simulink model "RobotX_FullSystemSep20"  (R2014a)
settings: Solver=FixedStepDiscrete  StartTime=0.0  StopTime=inf  FixedStep=.25  RelTol=1e-3
undefined symbols (not defined in the file): Com1, Com2, Com3, Com4, DiscIntNeverNeededParam, standard
libraries: simulink x11, xpcseriallib x11, slrtlib x3, speedgoatlib x1, speedgoatlib_IO102 x1
(part 2 of 4)

== matlab function RobotX_FullSystemSep20/Main FSM/Start//Speedgate/Start Gate/Calculate Times ==
  data: pts input; u input; Data output
function Data = calcTimes(pts, u)
%Written by Anderson Lebbad on August 9, 2014
%Last Edited:

%Calculates times for the boat to get to points for a trajectory, and
%formats Data for communication

%Initialize
Data = zeros(24,1);
traj = zeros(8,3);

pts8 = [pts(1,:); (pts(2,:)-pts(1,:))/3; 2*(pts(2,:)-pts(1,:))/3; pts(2,:);...
    (pts(3,:)-pts(2,:))/2; pts(3,:); (pts(4,:)-pts(3,:))/2; pts(4,:)];

traj(:,1:2) = pts8;

for k = 2:8
    %Calculate distance to travel from last point
    distTravel = sqrt(sum((pts8(k-1,:)-pts8(k,:)).^2));
    %Assume 1m per second speed
    traj(k,3) = traj(k-1,3) + distTravel;
    %Add time based off initial velocity to get to first point past initial
    if k == 2
        traj(k,3) = traj(k,3) + 2.5*abs(2-u);
    end
end


%Output Data
for i=1:8
    for j = 1:3
        Data(3*(i-1)+j) = traj(i,j);
    end
end

== matlab function RobotX_FullSystemSep20/Main FSM/Start//Speedgate/Start Gate/Gate ==
  data: HeldHeading input; Finished output; Valid output; X input; Y input; Psi input; Dist input; Angles input; pts output; idx input
function [Finished, Valid, pts] = Gate(HeldHeading,X,Y,Psi,Dist,Angles,idx)
%Written by Anderson Lebbad on August 9, 2014
%Last Edited by:

%This function sends a forward trajectory (from the initial heading read
%into it) until a landmark is found. Once the landmark is found, a
%trajectory is written to dodge around it.

persistent Found finPt sample
if isempty(Found)
    Found = 0;
    finPt = [0 0];
    sample = 50;
end

dodgeLength = 15;
dodgeWidth = 5;
Finished = 0;
Valid = 0;
pts = zeros(4,2);
%Distance to object in meters
DistM = Dist/100;

%Set Valid bit. If it has been found in a previous timestep, the point is
%invalid, otherwise it is valid every increment of ts or if an object is
%found

%If no Landmark is found, navigate forward
if Found == 0
    %Initial pt
    pts(1,1) = X + 5*cos(HeldHeading*pi/180);
    pts(1,2) = Y + 5*sin(HeldHeading*pi/180);
    %Nothing found
    if idx(1) == 0
        pts(2,1) = X + 10*cos(HeldHeading*pi/180);
        pts(2,2) = Y + 10*sin(HeldHeading*pi/180);
        pts(3,1) = X + 15*cos(HeldHeading*pi/180);
        pts(3,2) = Y + 15*sin(HeldHeading*pi/180);
        pts(4,1) = X + 20*cos(HeldHeading*pi/180);
        pts(4,2) = Y + 20*sin(HeldHeading*pi/180);
        %Only flip valid bit every ts (seconds)
        sample = sample + 1;
        if sample >= 50
            Valid = 1;
            sample = 0;
        end
        %Something found
    elseif idx(2) == 0
        %Absolute Heading of object relative to boat's position
        landmarkHeading = mod((Psi + Angles(idx(1))),360);
        lmHeadingRad = landmarkHeading*pi/180;
        %Navigate to it
        pts(2,1) = X + DistM(idx(1))*cos(lmHeadingRad) - dodgeWidth*sin(lmHeadingRad);
        pts(2,2) = Y + DistM(idx(1))*sin(lmHeadingRad) + dodgeWidth*cos(lmHeadingRad);
        pts(3,1) = X + (DistM(idx(1)) + dodgeLength)*cos(lmHeadingRad);
        pts(3,2) = Y + (DistM(idx(1)) + dodgeLength)*sin(lmHeadingRad);
        pts(4,1) = X + (DistM(idx(1)) + 2*dodgeLength)*cos(lmHeadingRad);
        pts(4,2) = Y + (DistM(idx(1)) + 2*dodgeLength)*sin(lmHeadingRad);
        finPt = pts(4,:);
        %Flip valid if found
        Valid = 1;
        %Tag object as having been found
        Found = 1;
    else
        %Absolute Heading of object relative to boat's position
        landmarkHeading1 = mod((Psi + Angles(idx(1))),360);
        lmHeadingRad1 = landmarkHeading1*pi/180;
        landmarkHeading2 = mod((Psi + Angles(idx(2))),360);
        lmHeadingRad2 = landmarkHeading2*pi/180;
        %Landmark locations in NED
        lmX1 = X + DistM(idx(1))*cos(lmHeadingRad1);
        lmY1 = Y + DistM(idx(1))*sin(lmHeadingRad1);
        lmX2 = X + DistM(idx(2))*cos(lmHeadingRad2);
        lmY2 = Y + DistM(idx(2))*sin(lmHeadingRad2);
        %Middle point
        midX = (lmX1 + lmX2) / 2;
        midY = (lmY1 + lmY2) / 2;
        %Navigate to it
        pts(2,1) = midX;
        pts(2,2) = midY;
        %Hold heading and continue from midpoint
        pts(3,1) = midX + 5*cos(HeldHeading*pi/180);
        pts(3,2) = midY + 5*sin(HeldHeading*pi/180);
        pts(4,1) = midX + 10*cos(HeldHeading*pi/180);
        pts(4,2) = midY + 10*sin(HeldHeading*pi/180);
        finPt = pts(4,:);
        %Flip valid if found
        Valid = 1;
        %Tag object as having been found
        Found = 2;
    end
end

if Found == 1
    if idx(2) ~= 0
        %Absolute Heading of object relative to boat's position
        landmarkHeading1 = mod((Psi + Angles(idx(1))),360);
        lmHeadingRad1 = landmarkHeading1*pi/180;
        landmarkHeading2 = mod((Psi + Angles(idx(2))),360);
        lmHeadingRad2 = landmarkHeading2*pi/180;
        %Landmark locations in NED
        lmX1 = X + DistM(idx(1))*cos(lmHeadingRad1);
        lmY1 = Y + DistM(idx(1))*sin(lmHeadingRad1);
        lmX2 = X + DistM(idx(2))*cos(lmHeadingRad2);
        lmY2 = Y + DistM(idx(2))*sin(lmHeadingRad2);
        %Middle point
        midX = (lmX1 + lmX2) / 2;
        midY = (lmY1 + lmY2) / 2;
        %Navigate to it
        pts(2,1) = midX;
        pts(2,2) = midY;
        %Hold heading and continue from midpoint
        pts(3,1) = midX + 5*cos(HeldHeading*pi/180);
        pts(3,2) = midY + 5*sin(HeldHeading*pi/180);
        pts(4,1) = midX + 10*cos(HeldHeading*pi/180);
        pts(4,2) = midY + 10*sin(HeldHeading*pi/180);
        finPt = pts(4,:);
        %Flip valid if found
        Valid = 1;
        %Tag object as having been found
        Found = 2;
    end
end

%Check to see how far the current pose is from the final point in the
%trajectory
if Found >= 1
range = abs(finPt(1)-X)+abs(finPt(2)-Y);
else
    range = 1000;
end
if range <= 5
    Finished = 1;
end

end

== matlab function RobotX_FullSystemSep20/Main FSM/Acoustic FSM/Drive Pt1/CalcTimes ==
  data: pts input; u input; Data output
function Data = calcTimes(pts, u)
%Written by Anderson Lebbad on August 9, 2014
%Last Edited: Dylan DeGaetano September 1, 2014

%Calculates times for the boat to get to points for a trajectory, and
%formats Data for communication

%Initialize
Data = zeros(24,1);
traj = zeros(8,3);
traj(:,1:2) = pts;



for k = 2:8
    %Calculate distance to travel from last point
    distTravel = sqrt(sum((pts(k-1,:)-pts(k,:)).^2));
    %Assume 1m per second speed
    traj(k,3) = traj(k-1,3) + distTravel;
    %Add time based off initial velocity to get to first point past initial
    if k == 2
        traj(k,3) = traj(k,3) + 2.5*abs(2-u);
    end
end


%Output Data
for i=1:8
    for j = 1:3
        Data(3*(i-1)+j) = traj(i,j);
    end
end

== matlab function RobotX_FullSystemSep20/Main FSM/Light Beacon/Approach/CalcTimes ==
  data: pts input; u input; Data output
function Data = calcTimes(pts, u)
%Written by Anderson Lebbad on August 9, 2014
%Last Edited: Dylan DeGaetano September 1, 2014

%Calculates times for the boat to get to points for a trajectory, and
%formats Data for communication

%Initialize
Data = zeros(24,1);
traj = zeros(8,3);
traj(:,1:2) = pts;



for k = 2:8
    %Calculate distance to travel from last point
    distTravel = sqrt(sum((pts(k-1,:)-pts(k,:)).^2));
    %Assume 1m per second speed
    traj(k,3) = traj(k-1,3) + distTravel;
    %Add time based off initial velocity to get to first point past initial
    if k == 2
        traj(k,3) = traj(k,3) + 2.5*abs(2-u);
    end
end


%Output Data
for i=1:8
    for j = 1:3
        Data(3*(i-1)+j) = traj(i,j);
    end
end

== matlab function RobotX_FullSystemSep20/Main FSM/Acoustic FSM/Drive Pt1/GPSMove ==
  data: X input; Finished output; valid output; Y input; Psi input; GoalPt input; pts output
function [Finished, valid, pts] = GPSmove(X,Y,Psi,GoalPt)
%Written by Dylan DeGaetano on September 1, 2014
%Last edited by: Michael Benson on September 4, 2014
%   Changed Sample to be a persistent variable so that pts will not be
%   recalculated every iteration.
%
%This function will go to a given NED cooridnate 



persistent Sample

if isempty(Sample)
    Sample = 0;
end

valid = 0;
Finished = 0;
pts = zeros(8,2);
%$Distance to object in meters

if Sample == 0
    valid = 1;
    pts(1,1) = X+5*cos(Psi*pi/180);
    pts(1,2) = Y+5*cos(Psi*pi/180);
    pts(8,1) = GoalPt(1,1);
    pts(8,2) = GoalPt(1,2);
    pts(2,:) = pts(1,:) +(1*(GoalPt-pts(1,:))/7);
    pts(3,:) = pts(1,:) +(2*(GoalPt-pts(1,:))/7);
    pts(4,:) = pts(1,:) +(3*(GoalPt-pts(1,:))/7);
    pts(5,:) = pts(1,:) +(4*(GoalPt-pts(1,:))/7);
    pts(6,:) = pts(1,:) +(5*(GoalPt-pts(1,:))/7);
    pts(7,:) = pts(1,:) +(6*(GoalPt-pts(1,:))/7);
    Sample = 1; 
else 
    range = sqrt(sum((GoalPt - [X Y]).^2));
    if range <= 3
        Finished = 1;
    end
end

== matlab function RobotX_FullSystemSep20/Main FSM/Light Beacon/Light Enabler ==
  data: taskSelector output; quadOut output; GPSEn output; SpinEn output; ApprchEn output; StareEn output; mainTask input; GPSFin input; SpinFin input; ApprchFin input; Found input
function [taskSelector,quadOut,GPSEn,SpinEn,ApprchEn,StareEn]=...
    Light_Enabler(mainTask,GPSFin,SpinFin,ApprchFin,Found)
%Written by Anderson Lebbad on July 19, 2013
%Last Edited: Dylan DeGaetano on September ,8 2014
%   Substring search for task was written in
%   Case switches were redundant, combined with first set of if statements
%
%Changes the value of MainMode and the enablers for the tasks within the
%Light Beacon FSM.
%Will loop through move and spin commands 5 times before terminating if
%nothing is found
persistent quad

if isempty (quad)
    quad = 0;
end


% Initialize enable signals
GPSEn = 0;
SpinEn = 0;
StareEn = 0;
ApprchEn = 0;

% Convert main task indicator to a string
mainTaskStr = char(mainTask);

% Adjust finished states based on user task selection (never skips
% initialization)
if ~isempty(strfind(mainTaskStr,'spin'))
    GPSFin = 1;
elseif ~isempty(strfind(mainTaskStr,'stare'))
    Found = 1;
end

%adjust finish states based on interation through loop
if (GPSFin == 1)&&(SpinFin == 1)&&(quad <=4)
    GPSFin = 0;
    quad = quad +1;
end

% Set enable signals based on state completion
if ApprchFin == 1;
    StareEn = 1;
    taskSelector = 4;
elseif Found == 1;
    ApprchEn = 1;
    taskSelector = 3;
elseif GPSFin == 0
    GPSEn = 1;
    taskSelector = 1;
else
    SpinEn = 1;
    taskSelector = 2;
end

quadOut = quad;

== matlab function RobotX_FullSystemSep20/Main FSM/Light Beacon/Stare/MATLAB Function ==
  data: X input; Data output; Y input; Psi input; Angles input; idx input; LidarMode output
function [Data,LidarMode] = Orient(X,Y,Psi,Angles,idx)
%Written by Dylan DeGaetano on September 2, 2014
%Last Edited:Dylan DeGaetano on September 10,2014

%This function passes the current pose data added to the angle of the Light 
%buoy This stare forces the Boat to stare at the bouy.This task must be in station 
%keeping mode

persistent holdPose Locked

if isempty(holdPose)
    holdPose = [X Y Psi];
    Locked = 0;
end

if Locked == 0
    if idx(1) ~= 0
        holdPose(3) = Psi + Angles(idx(1));
        Locked = 1;
    end
end

%Initialize Data variable
Data = zeros(24,1);

%Set desired pose
Data(1) = holdPose(1);
Data(2) = holdPose(2);
Data(3) = holdPose(3);

if Locked == 0
    LidarMode = 1;
else
    LidarMode = 7;
end

end

== matlab function RobotX_FullSystemSep20/Main FSM/Light Beacon/GPS Move/CalcTimes ==
  data: pts input; u input; Data output
function Data = calcTimes(pts, u)
%Written by Anderson Lebbad on August 9, 2014
%Last Edited: Dylan DeGaetano September 1, 2014

%Calculates times for the boat to get to points for a trajectory, and
%formats Data for communication

%Initialize
Data = zeros(24,1);
traj = zeros(8,3);
traj(:,1:2) = pts;



for k = 2:8
    %Calculate distance to travel from last point
    distTravel = sqrt(sum((pts(k-1,:)-pts(k,:)).^2));
    %Assume 1m per second speed
    traj(k,3) = traj(k-1,3) + distTravel;
    %Add time based off initial velocity to get to first point past initial
    if k == 2
        traj(k,3) = traj(k,3) + 2.5*abs(2-u);
    end
end


%Output Data
for i=1:8
    for j = 1:3
        Data(3*(i-1)+j) = traj(i,j);
    end
end

== matlab function RobotX_FullSystemSep20/Main FSM/Light Beacon/GPS Move/GPSMove ==
  data: GoalN input; GoalE input; X input; Finished output; valid output; Y input; Psi input; pts output
function [Finished,valid,pts] = GPSmove(GoalN,GoalE,X,Y,Psi)
%Written by Dylan DeGaetano on September 1, 2014
%Last edited by: Anderson Lebbad
%
%This function will go to a given NED cooridnate, last edit changed the
%goal pt and variable names

GoalNED = [GoalN GoalE];

persistent Sample
if isempty(Sample)
Sample = 0;
end
Finished = 0;
pts = zeros(8,2);
%$Distance to object in meters

if Sample == 0
    pts(1,1) = X+5*cos(Psi*pi/180);
    pts(1,2) = Y+5*cos(Psi*pi/180);
    pts(8,:) = GoalNED;
    pts(2,:) = pts(1,:) +(1*(GoalNED-pts(1,:))/7);
    pts(3,:) = pts(1,:) +(2*(GoalNED-pts(1,:))/7);
    pts(4,:) = pts(1,:) +(3*(GoalNED-pts(1,:))/7);
    pts(5,:) = pts(1,:) +(4*(GoalNED-pts(1,:))/7);
    pts(6,:) = pts(1,:) +(5*(GoalNED-pts(1,:))/7);
    pts(7,:) = pts(1,:) +(6*(GoalNED-pts(1,:))/7);
    Sample = 1; 
    valid = 1;
    
else 
    range = sqrt(sum((GoalNED - [X Y]).^2));
    if range <= 5
        Finished = 1;
    end
    valid = 0;
end

== matlab function RobotX_FullSystemSep20/Main FSM/Light Beacon/GPS Move/LLA to NED ==
  data: quad input; GoalLLA input; GoalN output; NED_origin input; GoalE output
function [GoalN, GoalE]  = LLA2NED(quad,GoalLLA,NED_origin)
%Written by Anderson Lebbad on September 20, 2014
%Last edited by:
%
%This function converts a target Latitude, Longitude, Altitude (LLA) point
%into North, East, Down (NED) coordinates

%First convert to earth centered, earth fixed frame
if quad == 0
    TargetLLA = sum(GoalLLA)./4;
else
    TargetLLA = GoalLLA(quad,:);
end

GoalECEF = lla2ecef([TargetLLA(1); TargetLLA(2); 0]);
%Then convert from ECEF to North East Down
GoalNEDvect = ecef2ned(NED_origin,GoalECEF);
GoalN = GoalNEDvect(1);
GoalE = GoalNEDvect(2);

end

function x_ecef = lla2ecef(x_lla)
% LLE2ECEF: Converts from geodetic latitude, longitude, and altitude to earth-centered earth-fixed Cartesian coordinates
% INPUT: latitude phi (rad), longitude lambda (rad), altitude h (m)
% OUTPUT: [x, y, z]' (m) earth-centered earth-fixed Cartesian coordinates
    a = 6378137; % equatorial radius of ellipsoid (semi-major axis) (m)
    b = 6356752; % polar axis radius of ellipsoid (semi-minor axis) (m)

    phi = x_lla(1);
    lambda = x_lla(2);
    h = x_lla(3);
    
    % auxiliar quantities f, e, and N
    f = (a-b)/a;
    e = f*(2-f);
    N = a/sqrt(1-(e*sin(phi))^2);
    x_ecef = [(N+h)*cos(phi)*cos(lambda); (N+h)*cos(phi)*sin(lambda); (N*(1-e^2)+h)*sin(phi)];
end

function [x_ned] = ecef2ned(ned_lla, x_ecef)
% ECEF2NED Converts from earth-centered, earth-fixed Cartesian coordinates to tangent plane
% INPUT:
% 1) x_ecef=[x,y,z]' (m) earth-centered, earth-fixed Cartesian coordinates
% 2) ned_lla=[phi,lambda]' consiting of latitude phi (rad), longitude lambda (rad) of NED origin
% OUTPUT:
% 1) x_ned=[x,y,z]' (m) in NED coordinate system with the origin [phi,lambda]'

    phi = ned_lla(1);
    lambda = ned_lla(2);

    % transformation  matrix
    T = [-sin(phi)*cos(lambda) -sin(phi)*sin(lambda)  cos(phi)
         -sin(lambda)           cos(lambda)           0
          cos(phi)*cos(lambda)   cos(phi)*sin(lambda)  sin(phi)];

     x_ned = T*(x_ecef-lla2ecef([phi, lambda, 0]')); % convert to NED
     x_ned(3) = -x_ned(3);
end

== matlab function RobotX_FullSystemSep20/Main FSM/Acoustic FSM/Main Enabler ==
  data: taskSelector output; Drive1En output; Acoustic1En output; Drive2En output; Drive1Fin input; Acoustic1Fin input; Drive2Fin input; Acoustic2Fin input; Drive3Fin input; Acoustic3Fin input; Acoustic2En output; Drive3En output; Acoustic3En output; PointEn output
function [taskSelector,Drive1En,Acoustic1En,Drive2En,Acoustic2En,Drive3En,...
    Acoustic3En,PointEn] = taskEnabler(Drive1Fin,Acoustic1Fin,Drive2Fin,...
    Acoustic2Fin,Drive3Fin,Acoustic3Fin)
%Written by Anderson Lebbad on July 19, 2013
%Last Edited: Edward Zhu on June 2, 2014
%   Substring search for task was written in
%   Case switches were redundant, combined with first set of if statements

%Changes the value of MainMode and the enablers for the tasks within the
%Main FSM.

% Initialize enable signals
Drive1En = 0;
Acoustic1En = 0;
Drive2En = 0;
Acoustic2En = 0;
Drive3En = 0;
Acoustic3En = 0;
PointEn = 0;

% Set enable signals based on state completion
if Drive1Fin == 0
    Drive1En = 1;
    taskSelector = 1;
elseif Acoustic1Fin == 0
    Acoustic1En = 1;
    taskSelector = 2;
elseif Drive2Fin == 0
    Drive2En = 1;
    taskSelector = 3;
elseif Acoustic2Fin == 0
    Acoustic2En = 1;
    taskSelector = 4;
elseif Drive3Fin == 0
    Drive3En = 1;
    taskSelector = 5;
elseif Acoustic3Fin == 0
    Acoustic3En = 1;
    taskSelector = 6;
else
    PointEn = 1;
    taskSelector = 7;
end

== matlab function RobotX_FullSystemSep20/Main FSM/Termination/CalcTimes ==
  data: pts input; u input; Data output
function Data = calcTimes(pts, u)
%Written by Anderson Lebbad on August 9, 2014
%Last Edited: Dylan DeGaetano September 1, 2014

%Calculates times for the boat to get to points for a trajectory, and
%formats Data for communication

%Initialize
Data = zeros(24,1);
traj = zeros(8,3);
traj(:,1:2) = pts;



for k = 2:8
    %Calculate distance to travel from last point
    distTravel = sqrt(sum((pts(k-1,:)-pts(k,:)).^2));
    %Assume 1m per second speed
    traj(k,3) = traj(k-1,3) + distTravel;
    %Add time based off initial velocity to get to first point past initial
    if k == 2
        traj(k,3) = traj(k,3) + 2.5*abs(2-u);
    end
end


%Output Data
for i=1:8
    for j = 1:3
        Data(3*(i-1)+j) = traj(i,j);
    end
end

== matlab function RobotX_FullSystemSep20/Main FSM/Termination/LLA to NED ==
  data: GoalLLA input; GoalNED output; NED_origin input
function GoalNED = LLA2NED(GoalLLA,NED_origin)
%Written by Anderson Lebbad on September 20, 2014
%Last edited by:
%
%This function converts a target Latitude, Longitude, Altitude (LLA) point
%into North, East, Down (NED) coordinates

%First convert to earth centered, earth fixed frame
GoalECEF = lla2ecef([GoalLLA, 0]');
%Then convert from ECEF to North East Down
GoalNEDvect = ecef2ned(NED_origin,GoalECEF);
GoalNED = GoalNEDvect(1:2)';

end

function x_ecef = lla2ecef(x_lla)
% LLE2ECEF: Converts from geodetic latitude, longitude, and altitude to earth-centered earth-fixed Cartesian coordinates
% INPUT: latitude phi (rad), longitude lambda (rad), altitude h (m)
% OUTPUT: [x, y, z]' (m) earth-centered earth-fixed Cartesian coordinates
    a = 6378137; % equatorial radius of ellipsoid (semi-major axis) (m)
    b = 6356752; % polar axis radius of ellipsoid (semi-minor axis) (m)

    phi = x_lla(1);
    lambda = x_lla(2);
    h = x_lla(3);
    
    % auxiliar quantities f, e, and N
    f = (a-b)/a;
    e = f*(2-f);
    N = a/sqrt(1-(e*sin(phi))^2);
    x_ecef = [(N+h)*cos(phi)*cos(lambda); (N+h)*cos(phi)*sin(lambda); (N*(1-e^2)+h)*sin(phi)];
end

function [x_ned] = ecef2ned(ned_lla, x_ecef)
% ECEF2NED Converts from earth-centered, earth-fixed Cartesian coordinates to tangent plane
% INPUT:
% 1) x_ecef=[x,y,z]' (m) earth-centered, earth-fixed Cartesian coordinates
% 2) ned_lla=[phi,lambda]' consiting of latitude phi (rad), longitude lambda (rad) of NED origin
% OUTPUT:
% 1) x_ned=[x,y,z]' (m) in NED coordinate system with the origin [phi,lambda]'

    phi = ned_lla(1);
    lambda = ned_lla(2);

    % transformation  matrix
    T = [-sin(phi)*cos(lambda) -sin(phi)*sin(lambda)  cos(phi)
         -sin(lambda)           cos(lambda)           0
          cos(phi)*cos(lambda)   cos(phi)*sin(lambda)  sin(phi)];

     x_ned = T*(x_ecef-lla2ecef([phi, lambda, 0]')); % convert to NED
     x_ned(3) = -x_ned(3);
end

== matlab function RobotX_FullSystemSep20/Main FSM/OD//OA Path/Calculate Times ==
  data: pts input; u input; Data output
function Data = calcTimes(pts, u)
%Written by Anderson Lebbad on August 9, 2014
%Last Edited:

%Calculates times for the boat to get to points for a trajectory, and
%formats Data for communication

%Initialize
Data = zeros(24,1);
traj = zeros(8,3);
traj(:,1:2) = pts;



for k = 2:8
    %Calculate distance to travel from last point
    distTravel = sqrt(sum((pts(k-1,:)-pts(k,:)).^2));
    %Assume 1m per second speed
    traj(k,3) = traj(k-1,3) + distTravel;
    %Add time based off initial velocity to get to first point past initial
    if k == 2
        traj(k,3) = traj(k,3) + 2.5*abs(2-u);
    end
end


%Output Data
for i=1:8
    for j = 1:3
        Data(3*(i-1)+j) = traj(i,j);
    end
end

== matlab function RobotX_FullSystemSep20/Main FSM/OD//OA Path/Map Grid (Held Length) ==
  data: exitGate input; relPose output; NEDcorners input; X input; Y input; Psi input; landmarks input; obGrid output; targetPt output; nodes output
function [relPose,obGrid,targetPt,nodes] = MapGridHeldLength(exitGate,...
    NEDcorners,X,Y,Psi,landmarks)
%Written By Anderson Lebbad on September 3, 2014
%Last Edited on:

%This function takes in the exit gate identifier, the converted coordinates
%(from GPS to NED) of the bounding box of the OD/OA task, the current pose
%and the landmark list from SLAM - and generates a grid, as well as
%relative location of the vessel and the exit gate in that grid for the A*
%planner. This grid is a fixed size, so the relative size of each region
%can vary slightly depending upon the size of the bounded region sent to
%it.

%% Convert SLAM landmarks to NED coordinates
valid = landmarks(:,1) ~= 0;
NEDlandmarks = [X+landmarks(valid,1)*cos(landmarks(valid,2)+Psi*pi/180),...
    Y+landmarks(valid,1)*sin(landmarks(valid,2)+Psi*pi/180)];

%% Create node map (conversion between grid coordinates and NED coordinates)

cells_vert = 25;
cells_horiz = 10;

%Create edge devisions - corners must be ordered. First row is the bottom
%left coordinate, then bottom right is second, followed by top left,
%and finally top right. Only need top and bottom, will segment vertically
%in loop
top_edge = (0:cells_horiz-1)'*...
    [(NEDcorners(4,1)-NEDcorners(3,1))/(cells_horiz-1) (NEDcorners(4,2)-NEDcorners(3,2))/(cells_horiz-1)]+...
    ones(cells_horiz,1)*NEDcorners(3,:);
bottom_edge = (0:1:cells_horiz-1)'*...
    [(NEDcorners(2,1)-NEDcorners(1,1))/(cells_horiz-1) (NEDcorners(2,2)-NEDcorners(1,2))/(cells_horiz-1)]+...
    ones(cells_horiz,1)*NEDcorners(1,:);

%Create node matrices, first layer is north value for that coordinate,
%second is east
nodes = zeros(cells_vert,cells_horiz,2);
for i=1:cells_vert
    for j=1:cells_horiz
        nodes(i,j,1) = (i-1)*(top_edge(j,1)-bottom_edge(j,1))/(cells_vert-1)+bottom_edge(j,1);
        nodes(i,j,2) = (i-1)*(top_edge(j,2)-bottom_edge(j,2))/(cells_vert-1)+bottom_edge(j,2);
    end
end

%Find closest grid point to vessel pose
[clist,rlist] = min(abs(nodes(:,:,1)-X)+abs(nodes(:,:,2)-Y));
[~,col] = min(clist);
row = rlist(col);
relPose = [row col];

%Find closest grid point to exit gate
exitPoint = (exitGate*2-1)*[(NEDcorners(4,1)-NEDcorners(3,1))/7 (NEDcorners(4,2)-NEDcorners(3,2))/7]+...
    NEDcorners(3,:);
[clist,rlist] = min(abs(nodes(:,:,1)-exitPoint(1))+abs(nodes(:,:,2)-exitPoint(2)));
[~,col] = min(clist);
row = rlist(col);
targetPt = [row col];

%% Populate obstacle grid

%Initialize obstacle grid size
obGrid = zeros(cells_vert,cells_horiz);

%Convert landmarks to NED coordinates
% NEDlandmarks = [(X+landmarks(:,1).*cos((Psi+landmarks(:,2))*pi/180)) (Y+landmarks(:,1).*sin((Psi+landmarks(:,2))*pi/180))];
%Find limits on north and east coordinates to remove landmarks from map
%that are from different tasks
Nmax = max(NEDcorners(:,1));
Nmin = min(NEDcorners(:,1));
Emax = max(NEDcorners(:,2));
Emin = min(NEDcorners(:,2));
%Mark landmarks out of bounded region
Nvalid = (NEDlandmarks(:,1)<Nmax & NEDlandmarks(:,1)>Nmin);
Evalid = (NEDlandmarks(:,2)<Emax & NEDlandmarks(:,2)>Emin);
NEbounded = Nvalid & Evalid;
NEDlandmarks(~NEbounded,:) = NaN;

%Relative coordinates for padding
neighbors_rel = [1,-1;1,0;1,1;0,1;-1,1;-1,0;-1,-1;0,-1];
%Find closest location for each of the landmarks in the obstacle grid
valid_landmark_idx = find(~isnan(NEDlandmarks(:,1)));
for q = 1:length(valid_landmark_idx)
    k = valid_landmark_idx(q);
    [clist,rlist] = min(abs(nodes(:,:,1)-NEDlandmarks(k,1))+abs(nodes(:,:,2)-NEDlandmarks(k,2)));
    [~,col] = min(clist);
    row = rlist(col);
    %Mark as obstacle
    obGrid(row,col) = -1;
    %Find grid coordinates for padding
    neighbors_abs = neighbors_rel + ones(8,1)*[row col];
    %Mark invalid indices
    neighbors_invalidX = (neighbors_abs(:,1)<=0) | (neighbors_abs(:,1)>cells_vert);
    neighbors_invalidY = (neighbors_abs(:,2)<=0) | (neighbors_abs(:,2)>cells_horiz);
    neighbors_invalid = neighbors_invalidX | neighbors_invalidY;
    neighbors_abs(neighbors_invalid,:) = NaN;
    %Track neighbors that are obstacles
    neighbors_obstacles = (obGrid(neighbors_abs(~neighbors_invalid,1)+...
        cells_vert*(neighbors_abs(~neighbors_invalid,2)-1)) == -1);
    neighbors_abs(neighbors_obstacles,:) = NaN;
    n_valid = ~isnan(neighbors_abs(:,1));
    %Flag padded area in obstacle grid, if already flagged, increase flag
    %val
    obGrid(neighbors_abs(n_valid,1)+cells_vert*(neighbors_abs(n_valid,2)-1)) = 2+...
        obGrid(neighbors_abs(n_valid,1)+cells_vert*(neighbors_abs(n_valid,2)-1));
end

end

== matlab function RobotX_FullSystemSep20/Main FSM/OD//OA Path/Path To Trajectory ==
  data: Finished output; time input; valid output; relPose input; trajectory output; Path input; nodes input
function [Finished,valid,trajectory]=PathToTrajectory(time,relPose,Path,nodes)
%Written By Anderson Lebbad on September 8, 2014

%This code takes the output path from the A*, the node map, and the
%relative pose of the vessel, and outputs a trajectory for the low level
%controller.

%% Initialize output
Finished = 0;
valid = 0;
trajectory = zeros(8,2);

%Time tracking variable for updating valid flag
persistent lastTime
if isempty(lastTime)
    lastTime = time - 5;
end

%% Determine grid points

num_on_path = sum(~isnan(Path(:,1)));
if num_on_path > 1
    
    %Find the closest location in the path to the current point
    [~,closestIdx] = min(abs(Path(:,1)-relPose(1))+abs(Path(:,2)-relPose(2)));
    
    %Find how many points there are past the initial in the path
    num_remaining = num_on_path - closestIdx + 1;
    
    %Find the last path point to pass
    if num_remaining > 8
        initIdx = closestIdx + 1;
        lastIdx = initIdx + 7;
        
        %Grab points
        points = Path(initIdx:lastIdx,:);
        
        %% Convert to NED and output
        
        %Find the NED coordinates of those grid points, and write output
        [m,n] = size(nodes(:,:,1));
        trajectory(:,1) = nodes(points(:,1)+m*(points(:,2)-1));
        trajectory(:,2) = nodes(points(:,1)+m*(points(:,2)-1)+m*n);
        %Check timing to flag valid
        timeDiff = time - lastTime;
        if timeDiff >= 5
            valid = 1;
            lastTime = time;
        end
    elseif num_remaining < 3
        Finished = 1;
    end
end

end

== matlab function RobotX_FullSystemSep20/Parameters/GPS Points/GPS Selector ==
  data: course input; ssGate output; ssGateA input; lightGPSA input; odoaCornerGPSA input; acouLocGPSA input; acouLocA input; dockA input; ssGateB input; lightGPSB input; odoaCornerGPSB input; acouLocGPSB input; acouLocB input; dockB input; ssGateT input; lightGPST input; odoaCornerGPST input; acouLocGPST input; acouLocT input; dockT input; lightGPS output; odoaCornerGPS output; obstNavEnd output; acouLoc output; dock output
function [ssGate,lightGPS,odoaCornerGPS,obstNavEnd,acouLoc,dock] = ...
    GPSselector(course,...
    ssGateA,lightGPSA,odoaCornerGPSA,acouLocGPSA,acouLocA,dockA,...
    ssGateB,lightGPSB,odoaCornerGPSB,acouLocGPSB,acouLocB,dockB,...
    ssGateT,lightGPST,odoaCornerGPST,acouLocGPST,acouLocT,dockT)

%Written by: Anderson Lebbad on July 18, 2013
%Last Edited: Edward Zhu on June
%   Data type mismatch addressed
%   Character conversion redundant

%Selects GPS Points to use based on input Course

%Check value of CourseStr and pass inputs accordingly

switch course
    case uint8('A')
        ssGate = ssGateA;
        lightGPS = lightGPSA;
        odoaCornerGPS = odoaCornerGPSA;
        obstNavEnd = acouLocGPSA;
        acouLoc = acouLocA;
        dock = dockA;
        
    case uint8('B')
        ssGate = ssGateB;
        lightGPS = lightGPSB;
        odoaCornerGPS = odoaCornerGPSB;
        obstNavEnd = acouLocGPSB;
        acouLoc = acouLocB;
        dock = dockB;
        
    otherwise
        ssGate = ssGateT;
        lightGPS = lightGPST;
        odoaCornerGPS = odoaCornerGPST;
        obstNavEnd = acouLocGPST;
        acouLoc = acouLocT;
        dock = dockT;
end

== system RobotX_FullSystemSep20/Main FSM/Light Beacon/Spin	 ==
  Sensors : Inport
  Enable : EnablePort  ShowOutputPort=on
  Bus Selector : BusSelector  OutputSignals=Navigation Message.Pose.X,Navigation Message.Pose.Y,Navigation Message.Pose.Psi,Lidar Data Input.Landmarks.Angles,Lidar Data Input.Color data.idx
  Compare To Constant : simulink/Logic and Bit Operations/Compare To Constant  relop=>=  const=10  OutDataTypeStr=boolean
  Data Type Conversion1 : DataTypeConversion  OutDataTypeStr=double
  Discrete-Time Integrator : DiscreteIntegrator  SampleTime=-1  ICPrevOutput=DiscIntNeverNeededParam  ICPrevScaledInput=DiscIntNeverNeededParam
  Logical Operator : Logic  Operator=OR  AllPortsSameDT=off  OutDataTypeStr=boolean
  Output Heirarchy : Subsystem
  Spin : MATLAB Function  TreatAsAtomicUnit=on
  Finished : Outport
  Outputs : Outport  Port=2
  Found : Outport  Port=3
  wires:
  Sensors/1 -> Output Heirarchy/2(Sensors), Bus Selector/1
  Bus Selector/1 -> Spin/2(X)  "<X>"
  Bus Selector/3 -> Spin/4(Psi)  "<Psi>"
  Bus Selector/2 -> Spin/3(Y)  "<Y>"
  Spin/2(Data) -> Output Heirarchy/1(Data)
  Output Heirarchy/1(Outputs) -> Outputs/1
  Enable/1 -> Discrete-Time Integrator/1
  Discrete-Time Integrator/1 -> Spin/1(time), Compare To Constant/1
  Spin/3(Found) -> Found/1
  Compare To Constant/1 -> Logical Operator/1
  Spin/1(Finished) -> Logical Operator/2
  Logical Operator/1 -> Data Type Conversion1/1
  Data Type Conversion1/1 -> Finished/1
  Bus Selector/4 -> Spin/5(Angles)  "<Angles>"
  Bus Selector/5 -> Spin/6(idx)  "<idx>"

== system RobotX_FullSystemSep20/Main FSM/Light Beacon/Stare ==
  note: Signal
  Sensors : Inport
  Enable : EnablePort  ShowOutputPort=on
  Bus Selector : BusSelector  OutputSignals=Navigation Message.Pose.X,Navigation Message.Pose.Y,Navigation Message.Pose.Psi,Lidar Data Input.Landmarks.Angles,Lidar Data Input.Color data.idx
  Compare To Constant : simulink/Logic and Bit Operations/Compare To Constant  relop=>=  const=45  OutDataTypeStr=boolean
  Data Type Conversion : DataTypeConversion  OutDataTypeStr=double
  Discrete-Time Integrator : DiscreteIntegrator  SampleTime=-1  ICPrevOutput=DiscIntNeverNeededParam  ICPrevScaledInput=DiscIntNeverNeededParam
  MATLAB Function : MATLAB Function  TreatAsAtomicUnit=on
  Output Heirarchy : Subsystem
  Finished : Outport
  Outputs : Outport  Port=2
  wires:
  Bus Selector/1 -> MATLAB Function/1(X)  "<X>"
  Discrete-Time Integrator/1 -> Compare To Constant/1
  Enable/1 -> Discrete-Time Integrator/1
  Compare To Constant/1 -> Data Type Conversion/1
  Data Type Conversion/1 -> Finished/1
  Sensors/1 -> Output Heirarchy/3(Sensors), Bus Selector/1
  Bus Selector/2 -> MATLAB Function/2(Y)  "<Y>"
  Bus Selector/3 -> MATLAB Function/3(Psi)  "<Psi>"
  MATLAB Function/1(Data) -> Output Heirarchy/1(Data)
  Output Heirarchy/1(Outputs) -> Outputs/1
  Bus Selector/4 -> MATLAB Function/4(Angles)  "<Angles>"
  Bus Selector/5 -> MATLAB Function/5(idx)  "<idx>"
  MATLAB Function/2(LidarMode) -> Output Heirarchy/2(Lidar Mode)

== system RobotX_FullSystemSep20/Main FSM/OD//OA Path/Output Reassign ==
  "Valid " : Inport
  Data : Inport  Port=2
  Sensors : Inport  Port=3
  Acoustic Active : Constant
  Bus Creator2 : BusCreator  Inputs=3
  Bus Creator3 : BusCreator  Inputs=3
  Bus Creator5 : BusCreator  Inputs=2
  Constant3 : Constant
  Lidar Mode : Constant  Value=3
  Outputs : Outport
  wires:
  Sensors/1 -> Bus Creator5/2  "Sensors"
  Bus Creator5/1 -> Outputs/1  "Output Signals"
  "Valid "/1 -> Bus Creator2/1  "Valid"
  Constant3/1 -> Bus Creator2/2  "Control Mode"
  Data/1 -> Bus Creator2/3  "Data"
  Bus Creator2/1 -> Bus Creator3/1  "Navigation Outputs"
  Acoustic Active/1 -> Bus Creator3/2  "Acoustic Active"
  Lidar Mode/1 -> Bus Creator3/3  "Lidar Mode"
  Bus Creator3/1 -> Bus Creator5/1  "Outputs"

== system RobotX_FullSystemSep20/Main FSM/RCHold/Direct Control ==
  Sensors : Inport
  Acoustic Active : Constant  Value=0
  Bus Creator2 : BusCreator  Inputs=3
  Bus Creator3 : BusCreator  Inputs=3
  Bus Creator4 : BusCreator  Inputs=2
  Constant : Constant
  Constant1 : Constant  Value=2
  Constant2 : Constant  Value=zeros(24,1)
  Lidar Mode : Constant  Value=3
  Outputs : Outport
  wires:
  Sensors/1 -> Bus Creator4/2  "Sensors"
  Bus Creator4/1 -> Outputs/1  "Output Signals"
  Bus Creator2/1 -> Bus Creator3/1  "Navigation Outputs"
  Acoustic Active/1 -> Bus Creator3/2  "Acoustic Active"
  Lidar Mode/1 -> Bus Creator3/3  "Lidar Mode"
  Bus Creator3/1 -> Bus Creator4/1  "Outputs"
  Constant/1 -> Bus Creator2/1  "Valid"
  Constant1/1 -> Bus Creator2/2  "Control Mode"
  Constant2/1 -> Bus Creator2/3  "Data"

== system RobotX_FullSystemSep20/Main FSM/Start//Speedgate/GPS Move ==
  Sensors : Inport
  Enable : EnablePort
  Bus Selector : BusSelector  OutputSignals=Navigation Message.Pose.X,Navigation Message.Pose.Y,Navigation Message.Pose.Psi,Navigation Message.Velocity.u
  CalcTimes : MATLAB Function  TreatAsAtomicUnit=on
  Data Store Read : DataStoreRead  DataStoreName=ssGateGPS
  Data Store Read1 : DataStoreRead  DataStoreName=NED_origin
  GPSMove : MATLAB Function  TreatAsAtomicUnit=on
  LLA to NED : MATLAB Function  TreatAsAtomicUnit=on
  Output Reassign : Subsystem
  Outputs : Outport
  Finished : Outport  Port=2
  wires:
  GPSMove/3(pts) -> CalcTimes/1(pts)
  Sensors/1 -> Output Reassign/3(Sensors), Bus Selector/1
  Bus Selector/1 -> GPSMove/2(X)  "<X>"
  Bus Selector/2 -> GPSMove/3(Y)  "<Y>"
  Bus Selector/3 -> GPSMove/4(Psi)  "<Psi>"
  Bus Selector/4 -> CalcTimes/2(u)  "<u>"
  GPSMove/1(Finished) -> Finished/1
  Output Reassign/1(Outputs) -> Outputs/1
  CalcTimes/1(Data) -> Output Reassign/2(Data)
  GPSMove/2(valid) -> Output Reassign/1(Vaild)
  LLA to NED/1(GoalNED) -> GPSMove/1(GoalNED)
  Data Store Read/1 -> LLA to NED/1(GoalLLA)
  Data Store Read1/1 -> LLA to NED/2(NED_origin)

== system RobotX_FullSystemSep20/Main FSM/Start//Speedgate/Speed Gate ==
  note: Through Gate
  Sensors : Inport
  Enable : EnablePort
  Bus Selector : BusSelector  OutputSignals=Navigation Message.Pose.X,Navigation Message.Pose.Y,Navigation Message.Pose.Psi,Lidar Data Input.Landmarks.Distances,Lidar Data Input.Landmarks.Angles,Lidar Data Input.Color data.idx,Navigation Message.Velocity.u
  Calculate Times : MATLAB Function  TreatAsAtomicUnit=on
  Data Store Read : DataStoreRead  DataStoreName=ssHeldHeading
  Gate : MATLAB Function  TreatAsAtomicUnit=on
  Output Reassign : Subsystem
  Outputs : Outport
  Finished : Outport  Port=2
  wires:
  Output Reassign/1(Outputs) -> Outputs/1
  Gate/1(Finished) -> Finished/1
  Sensors/1 -> Output Reassign/3(Sensors), Bus Selector/1
  Bus Selector/3 -> Gate/4(Psi)  "<Psi>"
  Bus Selector/2 -> Gate/3(Y)  "<Y>"
  Bus Selector/4 -> Gate/5(Dist)  "<Distances>"
  Bus Selector/5 -> Gate/6(Angles)  "<Angles>"
  Bus Selector/1 -> Gate/2(X)  "<X>"
  Bus Selector/7 -> Calculate Times/2(u)  "<u>"
  Gate/3(pts) -> Calculate Times/1(pts)
  Calculate Times/1(Data) -> Output Reassign/2(Data)
  Gate/2(Valid) -> Output Reassign/1(Vaild)
  Data Store Read/1 -> Gate/1(HeldHeading)
  Bus Selector/6 -> Gate/7(idx)  "<idx>"

== system RobotX_FullSystemSep20/Main FSM/Start//Speedgate/Start Gate ==
  note: Through Gate
  Sensors : Inport
  Enable : EnablePort
  Bus Selector : BusSelector  OutputSignals=Navigation Message.Pose.X,Navigation Message.Pose.Y,Navigation Message.Pose.Psi,Lidar Data Input.Landmarks.Distances,Lidar Data Input.Landmarks.Angles,Lidar Data Input.Color data.idx,Navigation Message.Velocity.u
  Calculate Times : MATLAB Function  TreatAsAtomicUnit=on
  Data Store Read : DataStoreRead  DataStoreName=ssHeldHeading
  Gate : MATLAB Function  TreatAsAtomicUnit=on
  Output Reassign : Subsystem
  Outputs : Outport
  Finished : Outport  Port=2
  wires:
  Output Reassign/1(Outputs) -> Outputs/1
  Gate/1(Finished) -> Finished/1
  Sensors/1 -> Output Reassign/3(Sensors), Bus Selector/1
  Bus Selector/3 -> Gate/4(Psi)  "<Psi>"
  Bus Selector/2 -> Gate/3(Y)  "<Y>"
  Bus Selector/4 -> Gate/5(Dist)  "<Distances>"
  Bus Selector/5 -> Gate/6(Angles)  "<Angles>"
  Bus Selector/1 -> Gate/2(X)  "<X>"
  Bus Selector/7 -> Calculate Times/2(u)  "<u>"
  Gate/3(pts) -> Calculate Times/1(pts)
  Calculate Times/1(Data) -> Output Reassign/2(Data)
  Gate/2(Valid) -> Output Reassign/1(Vaild)
  Data Store Read/1 -> Gate/1(HeldHeading)
  Bus Selector/6 -> Gate/7(idx)  "<idx>"

== system RobotX_FullSystemSep20/Main FSM/Termination/Output Reassign ==
  Vaild : Inport
  Data : Inport  Port=2
  Sensors : Inport  Port=3
  Acoustic Active : Constant  Value=0
  Bus Creator2 : BusCreator  Inputs=3
  Bus Creator3 : BusCreator  Inputs=3
  Bus Creator5 : BusCreator  Inputs=2
  Constant3 : Constant  Value=0
  Lidar Mode : Constant  Value=0
  Outputs : Outport
  wires:
  Sensors/1 -> Bus Creator5/2  "Sensors"
  Bus Creator5/1 -> Outputs/1  "Output Signals"
  Vaild/1 -> Bus Creator2/1  "Valid"
  Constant3/1 -> Bus Creator2/2  "Control Mode"
  Data/1 -> Bus Creator2/3  "Data"
  Bus Creator2/1 -> Bus Creator3/1  "Navigation Outputs"
  Acoustic Active/1 -> Bus Creator3/2  "Acoustic Active"
  Lidar Mode/1 -> Bus Creator3/3  "Lidar Mode"
  Bus Creator3/1 -> Bus Creator5/1  "Outputs"

== system RobotX_FullSystemSep20/Sensors/Serial In/ Raspberry Pi LCM (Acoustic) ==
  LCM Input : Inport
  ASCII Decode 6 : xpcseriallib/ASCII Decode   format=Deploy:%1u, Elapsed:%g, Bearing1:%g Bearing2:%g \r\n  nvars=4  vartypes={}
  Bus Creator : BusCreator  Inputs=2
  Bus Creator1 : BusCreator  Inputs=3
  FIFO ASCII read 1 : xpcseriallib/FIFO ASCII read   header={'Deploy:'}  term=[13 10]  hold=Zero output if no new data  enable=off  maxsize=1024  outputtype=8 bit uint null terminated  sampletime=-1
  LCM Output : Outport
  wires:
  LCM Input/1 -> FIFO ASCII read 1/1
  FIFO ASCII read 1/1 -> ASCII Decode 6/1
  ASCII Decode 6/3 -> Bus Creator/1  "Horizontal Bearing"
  ASCII Decode 6/4 -> Bus Creator/2  "Vertical Bearing"
  Bus Creator/1 -> Bus Creator1/3  "Bearings"
  ASCII Decode 6/2 -> Bus Creator1/2  "Elapsed Time"
  ASCII Decode 6/1 -> Bus Creator1/1  "Deployed"
  Bus Creator1/1 -> LCM Output/1  "Acoustic Message"

== system RobotX_FullSystemSep20/Sensors/Serial In/ Raspberry Pi LCM (Navigation) ==
  LCM Input : Inport
  ASCII Decode 6 : xpcseriallib/ASCII Decode   format=P1:%f P2:%f P3:%f V1:%f V2:%f V3:%f E1:%f E2:%f E3:%f Pt1:%f Pt2:%f St1:%f St2:%f Start:%f Elapsed:%f RC:%d \r\n  nvars=16  vartypes={}
  Bus Creator1 : BusCreator  Inputs=3
  Bus Creator2 : BusCreator  Inputs=3
  Bus Creator3 : BusCreator  Inputs=3
  Bus Creator4 : BusCreator  Inputs=8
  Bus Creator5 : BusCreator  Inputs=2
  Bus Creator6 : BusCreator  Inputs=2
  Data Type Conversion : DataTypeConversion  OutDataTypeStr=double
  FIFO ASCII read 1 : xpcseriallib/FIFO ASCII read   header={'P1:'}  term=[13 10]  hold=Zero output if no new data  enable=off  maxsize=1024  outputtype=8 bit uint null terminated  sampletime=-1
  LCM Output : Outport
  wires:
  LCM Input/1 -> FIFO ASCII read 1/1
  FIFO ASCII read 1/1 -> ASCII Decode 6/1
  Bus Creator4/1 -> LCM Output/1  "Navigation Message"
  ASCII Decode 6/1 -> Bus Creator1/1  "X"
  ASCII Decode 6/2 -> Bus Creator1/2  "Y"
  ASCII Decode 6/3 -> Bus Creator1/3  "Psi"
  Bus Creator1/1 -> Bus Creator4/1  "Pose"
  ASCII Decode 6/4 -> Bus Creator2/1  "u"
  ASCII Decode 6/5 -> Bus Creator2/2  "v"
  Bus Creator2/1 -> Bus Creator4/2  "Velocity"
  ASCII Decode 6/7 -> Bus Creator3/1  "Roll"
  ASCII Decode 6/8 -> Bus Creator3/2  "Pitch"
  ASCII Decode 6/9 -> Bus Creator3/3  "Yaw"
  Bus Creator3/1 -> Bus Creator4/3  "Euler"
  Bus Creator5/1 -> Bus Creator4/4  "Port"
  Bus Creator6/1 -> Bus Creator4/5  "Stbd"
  ASCII Decode 6/12 -> Bus Creator6/1  "StThrust"
  ASCII Decode 6/13 -> Bus Creator6/2  "StAzimuth"
  ASCII Decode 6/10 -> Bus Creator5/1  "PtThrust"
  ASCII Decode 6/11 -> Bus Creator5/2  "PtAzimuth"
  ASCII Decode 6/14 -> Bus Creator4/6  "Start"
  ASCII Decode 6/15 -> Bus Creator4/7  "Elapsed"
  ASCII Decode 6/16 -> Data Type Conversion/1  "On/Off/RC/Auto"
  Data Type Conversion/1 -> Bus Creator4/8  "On/Off/RC/Auto"
  ASCII Decode 6/6 -> Bus Creator2/3  "r"

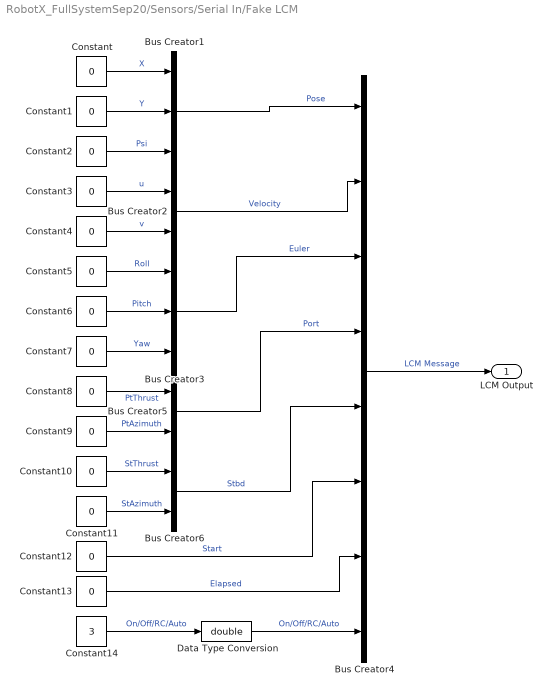
== system RobotX_FullSystemSep20/Sensors/Serial In/Fake LCM ==
  Bus Creator1 : BusCreator  Inputs=3
  Bus Creator2 : BusCreator  Inputs=2
  Bus Creator3 : BusCreator  Inputs=3
  Bus Creator4 : BusCreator  Inputs=8
  Bus Creator5 : BusCreator  Inputs=2
  Bus Creator6 : BusCreator  Inputs=2
  Constant{,1..13} (14 alike) : Constant  Value=0
  Constant14 : Constant  Value=3
  Data Type Conversion : DataTypeConversion  OutDataTypeStr=double
  LCM Output : Outport
  wires:
  Bus Creator4/1 -> LCM Output/1  "LCM Message"
  Constant/1 -> Bus Creator1/1  "X"
  Constant1/1 -> Bus Creator1/2  "Y"
  Constant2/1 -> Bus Creator1/3  "Psi"
  Bus Creator1/1 -> Bus Creator4/1  "Pose"
  Constant3/1 -> Bus Creator2/1  "u"
  Constant4/1 -> Bus Creator2/2  "v"
  Bus Creator2/1 -> Bus Creator4/2  "Velocity"
  Constant5/1 -> Bus Creator3/1  "Roll"
  Constant6/1 -> Bus Creator3/2  "Pitch"
  Constant7/1 -> Bus Creator3/3  "Yaw"
  Bus Creator3/1 -> Bus Creator4/3  "Euler"
  Bus Creator5/1 -> Bus Creator4/4  "Port"
  Bus Creator6/1 -> Bus Creator4/5  "Stbd"
  Constant10/1 -> Bus Creator6/1  "StThrust"
  Constant11/1 -> Bus Creator6/2  "StAzimuth"
  Constant8/1 -> Bus Creator5/1  "PtThrust"
  Constant9/1 -> Bus Creator5/2  "PtAzimuth"
  Constant12/1 -> Bus Creator4/6  "Start"
  Constant13/1 -> Bus Creator4/7  "Elapsed"
  Constant14/1 -> Data Type Conversion/1  "On/Off/RC/Auto"
  Data Type Conversion/1 -> Bus Creator4/8  "On/Off/RC/Auto"

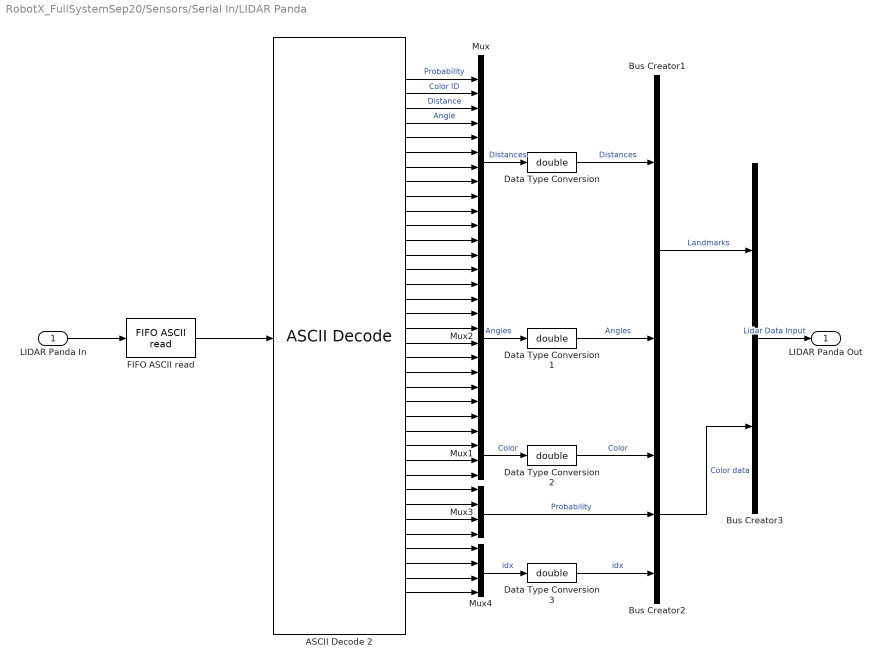
== system RobotX_FullSystemSep20/Sensors/Serial In/LIDAR Panda ==
  LIDAR Panda In : Inport
  ASCII Decode 2 : xpcseriallib/ASCII Decode   format=A:%d B:%d C:%d E:%d F:%d G:%d H:%d I:%d J:%d K:%d L:%d M:%d N:%d O:%d P:%d Q:%d R:%d S:%d T:%d U:%d V:%d W:%d X:%d C1:%d C2:%d C3:%d C4:%d P1:%f P2:%f P3:%f P4:%f I1:%d I2:%d I3:%d I4:%d \r\n  nvars=36  vartypes={}
  Bus Creator1 : BusCreator  Inputs=2
  Bus Creator2 : BusCreator  Inputs=3
  Bus Creator3 : BusCreator  Inputs=2
  Data Type Conversion{,1..3} (4 alike) : DataTypeConversion  OutDataTypeStr=double
  "FIFO ASCII read " : xpcseriallib/FIFO ASCII read   header={'A:'}  term=[13 10]  hold=Zero output if no new data  enable=off  maxsize=1024  outputtype=8 bit uint null terminated  sampletime=-1
  Mux : Mux  Inputs=12
  Mux1 : Mux
  Mux2 : Mux  Inputs=12
  Mux3 : Mux
  Mux4 : Mux
  LIDAR Panda Out : Outport
  wires:
  LIDAR Panda In/1 -> "FIFO ASCII read "/1
  "FIFO ASCII read "/1 -> ASCII Decode 2/1
  ASCII Decode 2/3 -> Mux/3  "Distance"
  ASCII Decode 2/2 -> Mux/2  "Color ID"
  ASCII Decode 2/4 -> Mux/4  "Angle"
  ASCII Decode 2/1 -> Mux/1  "Probability"
  ASCII Decode 2/7 -> Mux/7
  ASCII Decode 2/10 -> Mux/10
  ASCII Decode 2/11 -> Mux/11
  ASCII Decode 2/6 -> Mux/6
  ASCII Decode 2/8 -> Mux/8
  ASCII Decode 2/9 -> Mux/9
  ASCII Decode 2/12 -> Mux/12
  ASCII Decode 2/5 -> Mux/5
  ASCII Decode 2/13 -> Mux2/1
  ASCII Decode 2/15 -> Mux2/3
  ASCII Decode 2/22 -> Mux2/10
  ASCII Decode 2/23 -> Mux2/11
  ASCII Decode 2/17 -> Mux2/5
  ASCII Decode 2/18 -> Mux2/6
  ASCII Decode 2/14 -> Mux2/2
  ASCII Decode 2/24 -> Mux2/12
  ASCII Decode 2/20 -> Mux2/8
  ASCII Decode 2/19 -> Mux2/7
  ASCII Decode 2/21 -> Mux2/9
  ASCII Decode 2/16 -> Mux2/4
  ASCII Decode 2/25 -> Mux1/1
  ASCII Decode 2/28 -> Mux1/4
  ASCII Decode 2/26 -> Mux1/2
  ASCII Decode 2/27 -> Mux1/3
  ASCII Decode 2/30 -> Mux3/2
  ASCII Decode 2/31 -> Mux3/3
  ASCII Decode 2/32 -> Mux3/4
  ASCII Decode 2/29 -> Mux3/1
  ASCII Decode 2/36 -> Mux4/4
  ASCII Decode 2/34 -> Mux4/2
  ASCII Decode 2/35 -> Mux4/3
  ASCII Decode 2/33 -> Mux4/1
  Mux/1 -> Data Type Conversion/1  "Distances"
  Mux2/1 -> Data Type Conversion1/1  "Angles"
  Mux1/1 -> Data Type Conversion2/1  "Color"
  Mux3/1 -> Bus Creator2/2  "Probability"
  Mux4/1 -> Data Type Conversion3/1  "idx"
  Bus Creator1/1 -> Bus Creator3/1  "Landmarks"
  Bus Creator2/1 -> Bus Creator3/2  "Color data"
  Bus Creator3/1 -> LIDAR Panda Out/1  "Lidar Data Input"
  Data Type Conversion/1 -> Bus Creator1/1  "Distances"
  Data Type Conversion1/1 -> Bus Creator1/2  "Angles"
  Data Type Conversion2/1 -> Bus Creator2/1  "Color"
  Data Type Conversion3/1 -> Bus Creator2/3  "idx"

== system RobotX_FullSystemSep20/Main FSM/Acoustic FSM/Acoustics Pt1/Output Heirarchy ==
  Data : Inport
  Sensors : Inport  Port=2
  Acoustic Active : Constant
  Bus Creator2 : BusCreator  Inputs=3
  Bus Creator3 : BusCreator  Inputs=3
  Bus Creator5 : BusCreator  Inputs=2
  Constant : Constant
  Constant3 : Constant
  Lidar Mode : Constant
  Outputs : Outport
  wires:
  Sensors/1 -> Bus Creator5/2  "Sensors"
  Bus Creator5/1 -> Outputs/1  "Output Signals"
  Constant/1 -> Bus Creator2/1  "Valid"
  Constant3/1 -> Bus Creator2/2  "Control Mode"
  Data/1 -> Bus Creator2/3  "Data"
  Bus Creator2/1 -> Bus Creator3/1  "Navigation Outputs"
  Acoustic Active/1 -> Bus Creator3/2  "Acoustic Active"
  Lidar Mode/1 -> Bus Creator3/3  "Lidar Mode"
  Bus Creator3/1 -> Bus Creator5/1  "Outputs"

== system RobotX_FullSystemSep20/Main FSM/Acoustic FSM/Acoustics Pt2/Output Heirarchy ==
  Data : Inport
  Sensors : Inport  Port=2
  Acoustic Active : Constant
  Bus Creator2 : BusCreator  Inputs=3
  Bus Creator3 : BusCreator  Inputs=3
  Bus Creator5 : BusCreator  Inputs=2
  Constant : Constant
  Constant3 : Constant
  Lidar Mode : Constant
  Outputs : Outport
  wires:
  Sensors/1 -> Bus Creator5/2  "Sensors"
  Bus Creator5/1 -> Outputs/1  "Output Signals"
  Constant/1 -> Bus Creator2/1  "Valid"
  Constant3/1 -> Bus Creator2/2  "Control Mode"
  Data/1 -> Bus Creator2/3  "Data"
  Bus Creator2/1 -> Bus Creator3/1  "Navigation Outputs"
  Acoustic Active/1 -> Bus Creator3/2  "Acoustic Active"
  Lidar Mode/1 -> Bus Creator3/3  "Lidar Mode"
  Bus Creator3/1 -> Bus Creator5/1  "Outputs"

== system RobotX_FullSystemSep20/Main FSM/Acoustic FSM/Acoustics Pt3/Output Heirarchy ==
  Data : Inport
  Sensors : Inport  Port=2
  Acoustic Active : Constant
  Bus Creator2 : BusCreator  Inputs=3
  Bus Creator3 : BusCreator  Inputs=3
  Bus Creator5 : BusCreator  Inputs=2
  Constant : Constant
  Constant3 : Constant
  Lidar Mode : Constant
  Outputs : Outport
  wires:
  Sensors/1 -> Bus Creator5/2  "Sensors"
  Bus Creator5/1 -> Outputs/1  "Output Signals"
  Constant/1 -> Bus Creator2/1  "Valid"
  Constant3/1 -> Bus Creator2/2  "Control Mode"
  Data/1 -> Bus Creator2/3  "Data"
  Bus Creator2/1 -> Bus Creator3/1  "Navigation Outputs"
  Acoustic Active/1 -> Bus Creator3/2  "Acoustic Active"
  Lidar Mode/1 -> Bus Creator3/3  "Lidar Mode"
  Bus Creator3/1 -> Bus Creator5/1  "Outputs"

== system RobotX_FullSystemSep20/Main FSM/Acoustic FSM/Drive Pt1/Output Reassign ==
  "Valid " : Inport
  Data : Inport  Port=2
  Sensors : Inport  Port=3
  Acoustic Active : Constant
  Bus Creator2 : BusCreator  Inputs=3
  Bus Creator3 : BusCreator  Inputs=3
  Bus Creator5 : BusCreator  Inputs=2
  Constant3 : Constant
  Lidar Mode : Constant
  Outputs : Outport
  wires:
  Sensors/1 -> Bus Creator5/2  "Sensors"
  Bus Creator5/1 -> Outputs/1  "Output Signals"
  "Valid "/1 -> Bus Creator2/1  "Valid"
  Constant3/1 -> Bus Creator2/2  "Control Mode"
  Data/1 -> Bus Creator2/3  "Data"
  Bus Creator2/1 -> Bus Creator3/1  "Navigation Outputs"
  Acoustic Active/1 -> Bus Creator3/2  "Acoustic Active"
  Lidar Mode/1 -> Bus Creator3/3  "Lidar Mode"
  Bus Creator3/1 -> Bus Creator5/1  "Outputs"

== system RobotX_FullSystemSep20/Main FSM/Acoustic FSM/Drive Pt2/Output Reassign ==
  "Valid " : Inport
  Data : Inport  Port=2
  Sensors : Inport  Port=3
  Acoustic Active : Constant
  Bus Creator2 : BusCreator  Inputs=3
  Bus Creator3 : BusCreator  Inputs=3
  Bus Creator5 : BusCreator  Inputs=2
  Constant3 : Constant
  Lidar Mode : Constant
  Outputs : Outport
  wires:
  Sensors/1 -> Bus Creator5/2  "Sensors"
  Bus Creator5/1 -> Outputs/1  "Output Signals"
  "Valid "/1 -> Bus Creator2/1  "Valid"
  Constant3/1 -> Bus Creator2/2  "Control Mode"
  Data/1 -> Bus Creator2/3  "Data"
  Bus Creator2/1 -> Bus Creator3/1  "Navigation Outputs"
  Acoustic Active/1 -> Bus Creator3/2  "Acoustic Active"
  Lidar Mode/1 -> Bus Creator3/3  "Lidar Mode"
  Bus Creator3/1 -> Bus Creator5/1  "Outputs"
